simulink model "bu_abslut125_romvect_float"  (R2021b)
settings: Solver=VariableStepAuto  StartTime=0.0  StopTime=350  RelTol=1e-3
undefined symbols (not defined in the file or in its folder): figd2104, xcu250
libraries: hdlBasic x1696, vmcUtilities x1
(part 4 of 8)

== matlab function bu_abslut125_romvect_float/MATLAB Function1 ==
  data: x input; out output; y input
function out = fcn(x,y)
tmp1 = x.^2 + y.^2;
out = cordicsqrt(tmp1);

== matlab function bu_abslut125_romvect_float/MATLAB Function ==
  data: u input; y output; x input
function y = fcn(u,x)

y = immse(u,x);

== matlab function bu_abslut125_romvect_float/MATLAB Function2 ==
  data: x input; out output; y input
function out = fcn(x,y)
out = sqrt(x.^2 + y.^2);
